simulink model "Predictive_control_verification"  (R2024b)
settings: Solver=FixedStepAuto  StartTime=0.0  StopTime=20  FixedStep=1  RelTol=1e-3
values from neighbouring files (symbols this model uses):
  verification = [0 0 ... (first row only)    [Predictive_verification.m]
settings Model: Creator=mvseg  LastModifiedBy=mvseg

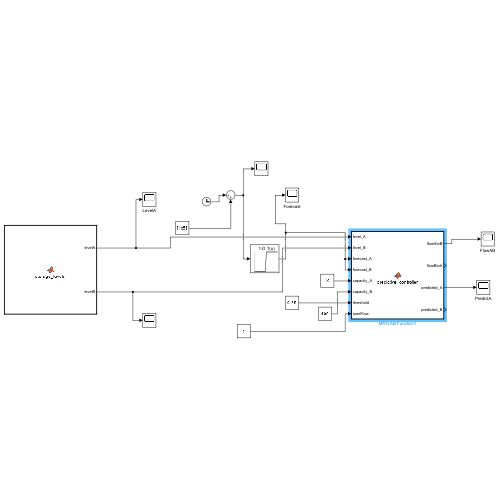
[thumbnail: Simulink's stored preview of the top-level diagram]
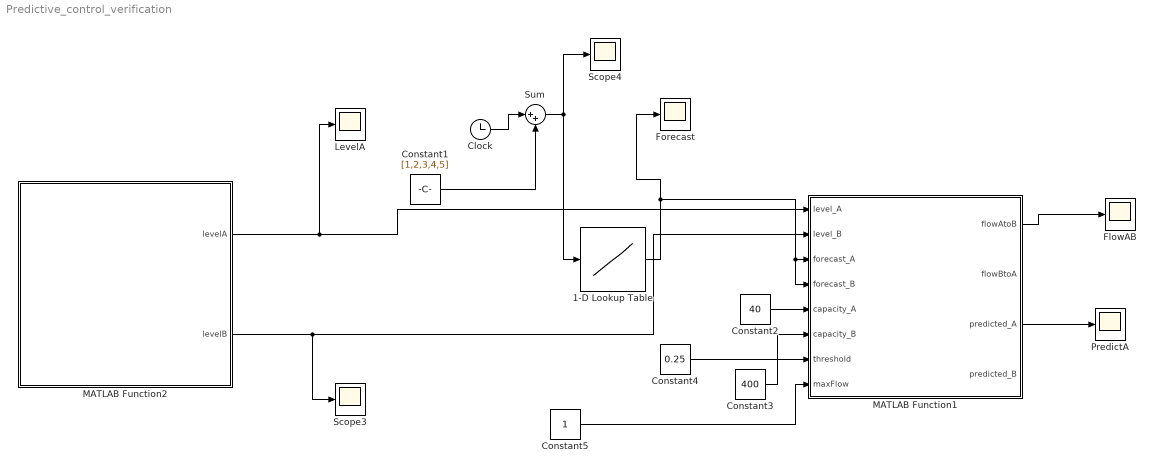
== system Predictive_control_verification ==
  1-D Lookup Table : Lookup_n-D  NumberOfTableDimensions=1  BreakpointsForDimension1=[0:19]  Table=verification(:,2)  InternalRulePriority=Speed  RndMeth=Simplest
  Clock : Clock
  Constant1 : Constant  Value=[1,2,3,4,5]
  Constant2 : Constant  Value=40
  Constant3 : Constant  Value=400
  Constant4 : Constant  Value=0.25
  Constant5 : Constant
  FlowAB : Scope
  Forecast : Scope
  LevelA : Scope
  MATLAB Function1 : MATLAB Function  TreatAsAtomicUnit=on
  MATLAB Function2 : MATLAB Function  TreatAsAtomicUnit=on
  PredictA : Scope
  Scope3 : Scope
  Scope4 : Scope
  Sum : Sum  Inputs=|++
  wires:
  Constant3/1 -> MATLAB Function1/6(capacity_B)
  MATLAB Function2/1(levelA) -> LevelA/1, MATLAB Function1/1(level_A)
  Constant5/1 -> MATLAB Function1/8(maxFlow)
  MATLAB Function2/2(levelB) -> Scope3/1, MATLAB Function1/2(level_B)
  Constant4/1 -> MATLAB Function1/7(threshold)
  Constant1/1 -> Sum/2
  Constant2/1 -> MATLAB Function1/5(capacity_A)
  1-D Lookup Table/1 -> MATLAB Function1/4(forecast_B), MATLAB Function1/3(forecast_A), Forecast/1
  Clock/1 -> Sum/1
  Sum/1 -> 1-D Lookup Table/1, Scope4/1
  MATLAB Function1/1(flowAtoB) -> FlowAB/1
  MATLAB Function1/3(predicted_A) -> PredictA/1

== matlab function Predictive_control_verification/MATLAB Function1 ==
  data: level_A input; level_B input; forecast_A input; flowAtoB output; forecast_B input; capacity_A input; capacity_B input; threshold input; maxFlow input; flowBtoA output; predicted_A output; predicted_B output
function [flowAtoB, flowBtoA, predicted_A, predicted_B] = ...
    predictive_controller(level_A, level_B, ...
                          forecast_A, forecast_B, ...
                          capacity_A, capacity_B, ...
                          threshold, maxFlow)

    % Initialize
    predicted_A = zeros(5,1);
    predicted_B = zeros(5,1);

    % Compute threshold levels in m^3
    threshold_level_A = threshold * capacity_A;
    threshold_level_B = threshold * capacity_B;

    % Predict levels
    for i = 1:5
        predicted_A(i) = level_A + sum(forecast_A(1:i));
        predicted_B(i) = level_B + sum(forecast_B(1:i));
    end

    % Get worst-case predicted levels
    max_predicted_A = max(predicted_A);
    max_predicted_B = max(predicted_B);

    % Compute overflow amounts (above threshold)
    overflow_A = max(max_predicted_A - threshold_level_A, 0);
    overflow_B = max(max_predicted_B - threshold_level_B, 0);

    % Safety check: do not allow transfer if the other tank would exceed threshold
    will_A_overflow = max_predicted_A >= threshold_level_A;
    will_B_overflow = max_predicted_B >= threshold_level_B;

    % Define a buffer margin to scale flows (e.g. 10% of capacity)
    bufferA = 0.9 * capacity_A;
    bufferB = 0.9 * capacity_B;

    % Control logic
    if overflow_A > 0 && ~will_B_overflow
        % Proportional transfer from A → B
        flowAtoB = min(maxFlow, maxFlow * (overflow_A / bufferA));
        flowBtoA = 0;
    elseif overflow_B > 0 && ~will_A_overflow
        % Proportional transfer from B → A
        flowBtoA = min(maxFlow, maxFlow * (overflow_B / bufferB));
        flowAtoB = 0;
    else
        flowAtoB = 0;
        flowBtoA = 0;
    end
end

== matlab function Predictive_control_verification/MATLAB Function2 ==
  data: levelA output; levelB output
function [levelA, levelB] = storage_levels()
    % Define persistent variables to keep track of levels
    persistent a b

    if isempty(a)
        a = 0; % Initial level A
    end
    if isempty(b)
        b = 0; % Initial level B
    end

    % Output current levels
    levelA = a;
    levelB = b;

    % Update for next timestep
    a = a + 1;     % A increases by 1
    b = b + 0.5;   % B increases by 0.5
end
